simulink model "flexibleDrive_NotchLead"  (R2021b)
settings: Solver=ode4  StartTime=0.0  StopTime=4  FixedStep=Ts  RelTol=1e-3  EnableMultiTasking=on
values from neighbouring files (symbols this model uses):
  b1 = 0.0257    [load_trajectory.m]
  b2 = 0.0026    [load_trajectory.m]
  C = 0    [load_trajectory.m]
  d1 = 0.5431    [load_trajectory.m]
  d2 = 0.0543    [load_trajectory.m]
  k = 0.025    [load_trajectory.m]
  m1 = 0.00031231    [load_trajectory.m]
  m2 = 0.00016865    [load_trajectory.m]
libraries: simulink x3
settings Model: Creator=user  LastModifiedBy=MTE360
settings SolverCC: AlgebraicLoopSolver=TrustRegion
settings DataIOCC: ReturnWorkspaceOutputs=off
settings OptimizationCC: LifeSpan=inf
settings DebuggingCC: SFUnexpectedBacktrackingDiag=warning  SFNoUnconditionalDefaultTransitionDiag=warning  SFMachineParentedDataDiag=warning  ArithmeticOperatorsInVariantConditions=warning
settings SFSimCC: SimUseLocalCustomCode=off  CustomCodeUndefinedFunction=UseInterfaceOnly
settings RTWCC: RTWUseLocalCustomCode=off
settings CodeAppCC: StateflowObjectComments=on
settings GRTTargetCC: TargetLangStandard=C89/C90 (ANSI)
settings ConfigComp: CovMetricSettings=dw  CovSaveCumulativeToWorkspaceVar=on  CovSaveSingleToWorkspaceVar=on  CovExternalEMLEnable=off

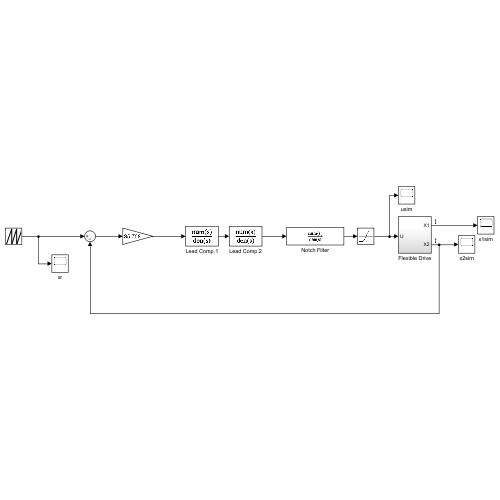
[thumbnail: Simulink's stored preview of the top-level diagram]
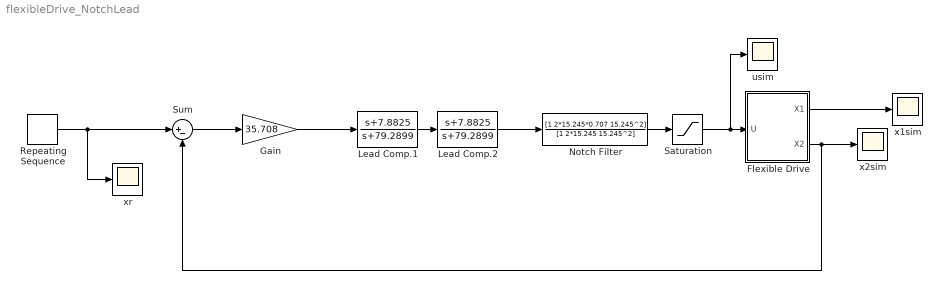
== system flexibleDrive_NotchLead ==
  Flexible Drive : Subsystem
  Gain : Gain  Gain=35.708
  Lead Comp.1 : TransferFcn  Numerator=[1 7.8825]  Denominator=[1 79.2899]
  Lead Comp.2 : TransferFcn  Numerator=[1 7.8825]  Denominator=[1 79.2899]
  Notch Filter : TransferFcn  Numerator=[1 2*15.245*0.707 15.245^2]  Denominator=[1 2*15.245 15.245^2]
  Repeating Sequence : simulink/Sources/Repeating Sequence  rep_seq_t=time  rep_seq_y=s
  Saturation : Saturate  UpperLimit=8  LowerLimit=-8
  Sum : Sum  Inputs=|+-
  usim : Scope
  x1sim : Scope
  x2sim : Scope
  xr : Scope
  wires:
  Flexible Drive/1(X1) -> x1sim/1
  Sum/1 -> Gain/1
  Flexible Drive/2(X2) -> x2sim/1, Sum/2
  Lead Comp.1/1 -> Lead Comp.2/1
  Gain/1 -> Lead Comp.1/1
  Repeating Sequence/1 -> xr/1, Sum/1
  Notch Filter/1 -> Saturation/1
  Lead Comp.2/1 -> Notch Filter/1
  Saturation/1 -> usim/1, Flexible Drive/1(U)

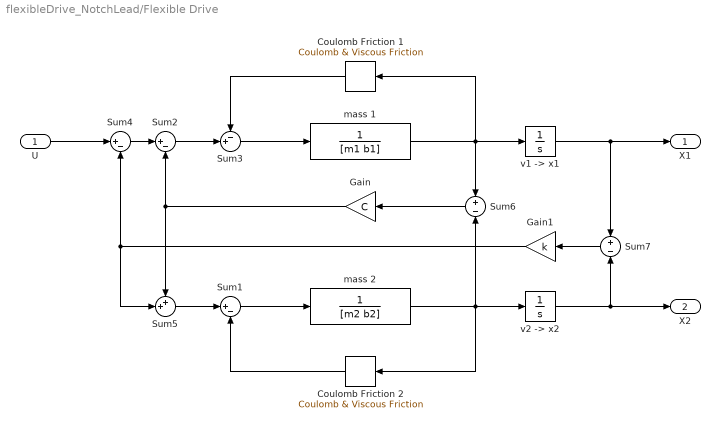
== system flexibleDrive_NotchLead/Flexible Drive ==
  U : Inport
  Coulomb Friction 1 : simulink/Discontinuities/Coulomb & Viscous Friction  offset=[d1]  gain=0
  Coulomb Friction 2 : simulink/Discontinuities/Coulomb & Viscous Friction  offset=[d2]  gain=0
  Gain : Gain  Gain=C  SaturateOnIntegerOverflow=on  OutDataTypeStr=Inherit: Same as input  ParamDataTypeStr=Inherit: Same as input
  Gain1 : Gain  Gain=k  SaturateOnIntegerOverflow=on  OutDataTypeStr=Inherit: Same as input  ParamDataTypeStr=Inherit: Same as input
  Sum1 : Sum  Inputs=|+-  SaturateOnIntegerOverflow=on
  Sum2 : Sum  Inputs=|+-  SaturateOnIntegerOverflow=on
  Sum3 : Sum  Inputs=-+|  SaturateOnIntegerOverflow=on
  Sum4 : Sum  Inputs=|+-  SaturateOnIntegerOverflow=on
  Sum5 : Sum  Inputs=++|  SaturateOnIntegerOverflow=on
  Sum6 : Sum  Inputs=+|-  SaturateOnIntegerOverflow=on
  Sum7 : Sum  Inputs=+|-  SaturateOnIntegerOverflow=on
  mass 1 : TransferFcn  Denominator=[m1 b1]
  mass 2 : TransferFcn  Denominator=[m2 b2]
  "v1 -> x1" : Integrator
  "v2 -> x2" : Integrator
  X1 : Outport  VectorParamsAs1DForOutWhenUnconnected=off
  X2 : Outport  Port=2  VectorParamsAs1DForOutWhenUnconnected=off
  wires:
  Sum3/1 -> mass 1/1
  Sum1/1 -> mass 2/1
  Sum2/1 -> Sum3/2
  Sum6/1 -> Gain/1
  Gain/1 -> Sum2/2, Sum5/1
  "v1 -> x1"/1 -> Sum7/1, X1/1
  "v2 -> x2"/1 -> X2/1, Sum7/2
  Sum7/1 -> Gain1/1
  Gain1/1 -> Sum4/2, Sum5/2
  Sum4/1 -> Sum2/1
  U/1 -> Sum4/1
  mass 2/1 -> "v2 -> x2"/1, Coulomb Friction 2/1, Sum6/2
  Sum5/1 -> Sum1/1
  Coulomb Friction 1/1 -> Sum3/1
  mass 1/1 -> "v1 -> x1"/1, Coulomb Friction 1/1, Sum6/1
  Coulomb Friction 2/1 -> Sum1/2
